simulink model "UAV_NL"  (R2016b)
settings: Solver=VariableStepAuto  StartTime=0.0  StopTime=300  FixedStep=SampleTime  RelTol=1e-3
InitFcn:
  | set_param('UAV_NL/Aircraft Model/Environment Model/Winds','BlockChoice','Wind Bypass');
  | set_param('UAV_NL/Aircraft Model/Environment Model/Magnetic Model','BlockChoice','WMM Bypass');
libraries: AircraftModel x1
settings Model: Creator=Paul Freeman  LastModifiedBy=UAVLAB
settings DataIOCC: SignalLoggingSaveFormat=ModelDataLogs  SaveState=on
settings OptimizationCC: ExpressionDepthLimit=2147483647  LifeSpan=inf
settings DebuggingCC: AlgebraicLoopMsg=none  SaveWithParameterizedLinksMsg=none  UnderspecifiedInitializationDetection=Classic  MergeDetectMultiDrivingBlocksExec=none  FcnCallInpInsideContextMsg=warning  UnconnectedInputMsg=none  UnconnectedOutputMsg=none  UnconnectedLineMsg=none  ModelReferenceExtraNoncontSigs=none  StateNameClashWarn=warning  SFUnexpectedBacktrackingDiag=warning  SFNoUnconditionalDefaultTransitionDiag=warning  SFExecutionAtInitializationDiag=none
settings HardwareCC: ProdBitPerPointer=32  ProdBitPerSizeT=32  ProdBitPerPtrDiffT=32  ProdLargestAtomicFloat=None  ProdIntDivRoundTo=Undefined  ProdEndianess=Unspecified  ProdWordSize=32  ProdHWDeviceType=32-bit Generic
settings ModelReferenceCC: PropagateSignalLabelsOutOfModel=off
settings GRTTargetCC: TargetLangStandard=C89/C90 (ANSI)  GeneratePreprocessorConditionals=Disable all  CombineOutputUpdateFcns=off  GRTInterface=on
settings ConfigComp: CovMetricSettings=dw  CovHtmlReporting=on  CovSaveCumulativeToWorkspaceVar=on  CovSaveSingleToWorkspaceVar=on  CovExternalEMLEnable=off  CovSFcnEnable=off

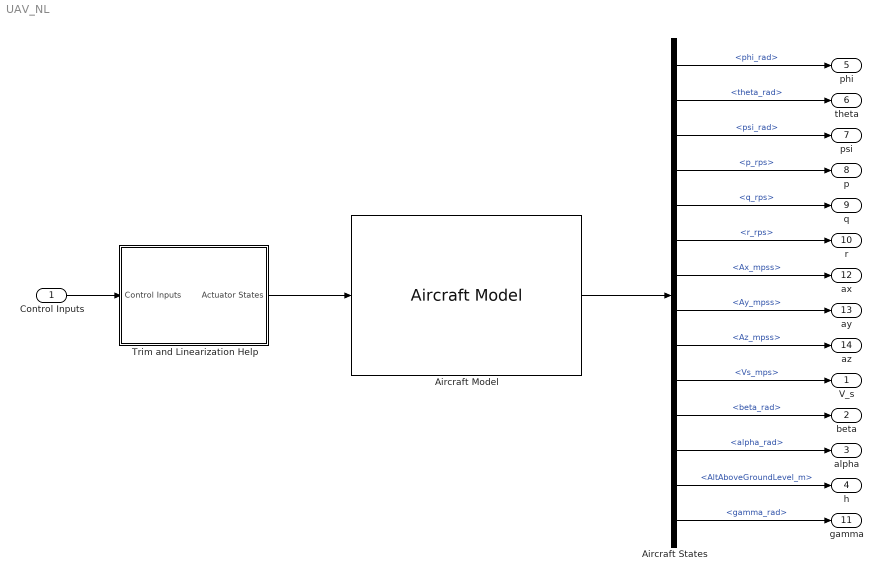
== system UAV_NL ==
  Control Inputs : Inport
  Aircraft Model : AircraftModel/Aircraft Model
  Aircraft States : BusSelector  OutputSignals=RigidStates.Euler.phi_rad,RigidStates.Euler.theta_rad,RigidStates.Euler.psi_rad,RigidStates.AngVel.p_rps,RigidStates.AngVel.q_rps,RigidStates.AngVel.r_rps,RigidStates.Accels.Ax_mpss,RigidStates.Accels.Ay_mpss,RigidStates.Accels.Az_mpss,AuxVar.WindAxesParams.Vs_mps,AuxVar.WindAxesParams.beta_rad,AuxVar.WindAxesParams.alpha_rad,AuxVar.Nav.AltAboveGroundLevel_m,AuxVar.Nav.gamma_rad
  Trim and Linearization Help : Subsystem
  V_s : Outport
  beta : Outport  Port=2
  alpha : Outport  Port=3
  h : Outport  Port=4
  phi : Outport  Port=5
  theta : Outport  Port=6
  psi : Outport  Port=7
  p : Outport  Port=8
  q : Outport  Port=9
  r : Outport  Port=10
  gamma : Outport  Port=11
  ax : Outport  Port=12
  ay : Outport  Port=13
  az : Outport  Port=14
  wires:
  Aircraft Model/1 -> Aircraft States/1
  Aircraft States/1 -> phi/1  "<phi_rad>"
  Aircraft States/2 -> theta/1  "<theta_rad>"
  Aircraft States/3 -> psi/1  "<psi_rad>"
  Aircraft States/4 -> p/1  "<p_rps>"
  Aircraft States/5 -> q/1  "<q_rps>"
  Aircraft States/6 -> r/1  "<r_rps>"
  Aircraft States/7 -> ax/1  "<Ax_mpss>"
  Aircraft States/8 -> ay/1  "<Ay_mpss>"
  Aircraft States/9 -> az/1  "<Az_mpss>"
  Aircraft States/10 -> V_s/1  "<Vs_mps>"
  Aircraft States/12 -> alpha/1  "<alpha_rad>"
  Aircraft States/14 -> gamma/1  "<gamma_rad>"
  Aircraft States/13 -> h/1  "<AltAboveGroundLevel_m>"
  Aircraft States/11 -> beta/1  "<beta_rad>"
  Control Inputs/1 -> Trim and Linearization Help/1(Control Inputs)
  Trim and Linearization Help/1(Actuator States) -> Aircraft Model/1

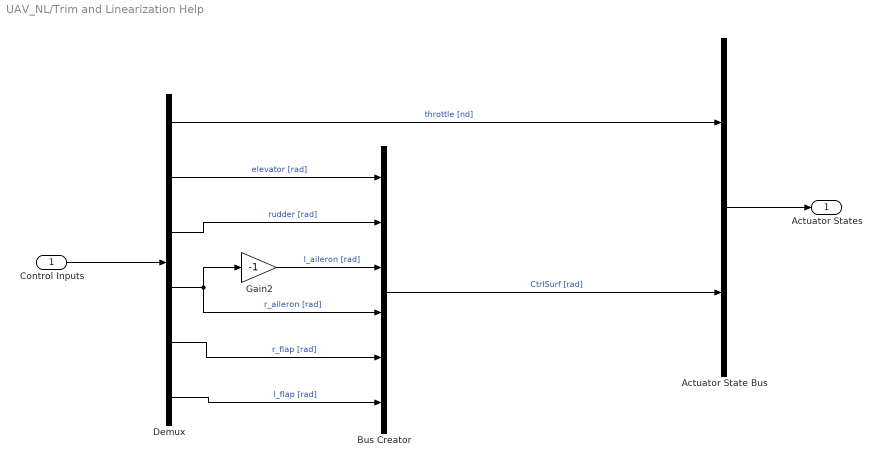
== system UAV_NL/Trim and Linearization Help ==
  Control Inputs : Inport
  Actuator State Bus : BusCreator  Inputs=2  OutDataTypeStr=Bus: Actuators
      settings: InheritFromInputs=off
  Bus Creator : BusCreator  Inputs=6
  Demux : Demux  Outputs=6
  Gain2 : Gain  Gain=-1
  Actuator States : Outport  OutDataTypeStr=Bus: Actuators
  wires:
  Demux/1 -> Actuator State Bus/1  "throttle [nd]"
  Demux/3 -> Bus Creator/2  "rudder [rad]"
  Demux/2 -> Bus Creator/1  "elevator [rad]"
  Bus Creator/1 -> Actuator State Bus/2  "CtrlSurf [rad]"
  Control Inputs/1 -> Demux/1
  Demux/5 -> Bus Creator/5  "r_flap [rad]"
  Demux/6 -> Bus Creator/6  "l_flap [rad]"
  Demux/4 -> Bus Creator/4, Gain2/1  "r_aileron [rad]"
  Gain2/1 -> Bus Creator/3  "l_aileron [rad]"
  Actuator State Bus/1 -> Actuator States/1
